simulink model "three_H_bridge"  (R2022b)
settings: Solver=FixedStepAuto  StartTime=0.0  StopTime=0.1  FixedStep=1e-7  MaxStep=1e-6  RelTol=5e-6
InitFcn:
  | fs=5000;
  | t1=(1/(3*fs));%模块内的载波时延
  | t2=(2/(3*fs));
  | m=1;
libraries: spsMosfetLib x72, spsSeriesRLCBranchLib x48, spsVoltageMeasurementLib x19, simulink x18, spsDCVoltageSourceLib x18, sps_lib x1
(part 1 of 2)
settings Model: Creator=zqf  LastModifiedBy=zqf

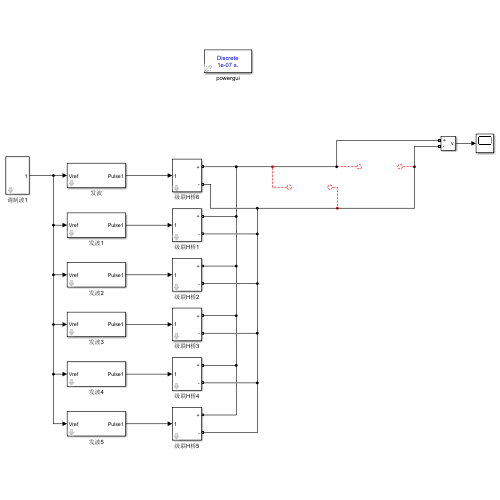
[thumbnail: Simulink's stored preview of the top-level diagram]
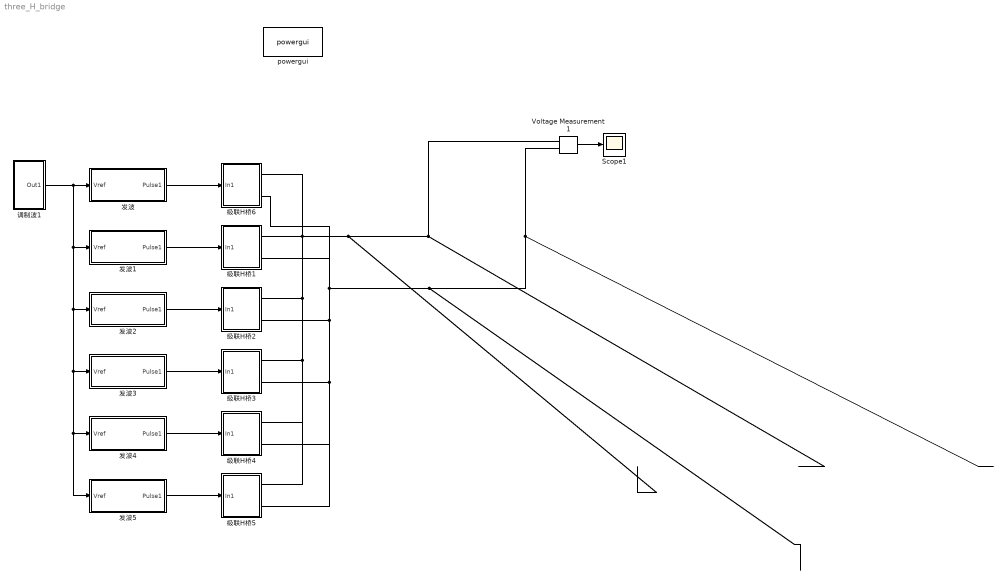
== system three_H_bridge ==
  Scope1 : Scope
  Voltage Measurement1 : spsVoltageMeasurementLib/Voltage Measurement  PhasorSimulation=off  OutputType=Complex  PSBequivalent=0
  powergui : sps_lib/powergui  Priority=1  SimulationMode=Discrete  SampleTime=1e-7  frequency=60  Iterations=50  frequencyindice=0  Pbase=100e6  ErrMax=1e-4  UnitsV=kV  UnitsW=MW  buscounter=0  FunctionMessages=off  echomessages=off  EnableUseOfTLC=off  CurrentSourceSwitches=off  DisableSnubberDevices=off  DisableRonSwitches=off  DisableVfSwitches=off  DisplayEquations=off  AutomaticDiscreteSolvers=off  SolverType=Tustin/Backward Euler (TBE)  Interpol=off  ExternalGateDelay=off  methode=off  Ts=100  x0status=blocks  SPID=on  SwTol=0  HookPort=off  NonlinearTolerance=1e-4  nMaxIteration=100  ContinueOnMaxIteration=off  RestoreLinks=warning  ResistiveCurrentMeasurement=off  Frange=[0:2:500]  Ylog=off  Xlog=on  ShowGrid=off  save=off  variable=ZData  structure=0  ZoomFFT=off  StartTime=0.0  cycles=1  DisplayStyle=1  fundamental=60  FreqAxis=off  MaxFrequency=1000  frequencyindicesteady=1  RmsSteady=1  display=off
  发波 : Subsystem  mask{n=0}
      mask prompts: n "延时n*Ts"
      mask DialogControl ParameterGroupVar Prompt: 参数
  发波1 : Subsystem  mask{n=(1/3)*(1/6)*m}
      mask prompts: n "延时n*Ts"
      mask DialogControl ParameterGroupVar Prompt: 参数
  发波2 : Subsystem  mask{n=(1/3)*(2/6)*m}
      mask prompts: n "延时n*Ts"
      mask DialogControl ParameterGroupVar Prompt: 参数
  发波3 : Subsystem  mask{n=(1/3)*(3/6)*m}
      mask prompts: n "延时n*Ts"
      mask DialogControl ParameterGroupVar Prompt: 参数
  发波4 : Subsystem  mask{n=(1/3)*(4/6)*m}
      mask prompts: n "延时n*Ts"
      mask DialogControl ParameterGroupVar Prompt: 参数
  发波5 : Subsystem  mask{n=(1/3)*(5/6)*m}
      mask prompts: n "延时n*Ts"
      mask DialogControl ParameterGroupVar Prompt: 参数
  级联H桥1 : Subsystem  mask{L=14E-6}
      mask DialogControl ParameterGroupVar Prompt: 参数
  级联H桥2 : Subsystem  mask{L=14E-6}
      mask DialogControl ParameterGroupVar Prompt: 参数
  级联H桥3 : Subsystem  mask{L=14E-6}
      mask DialogControl ParameterGroupVar Prompt: 参数
  级联H桥4 : Subsystem  mask{L=14E-6}
      mask DialogControl ParameterGroupVar Prompt: 参数
  级联H桥5 : Subsystem  mask{L=14E-6}
      mask DialogControl ParameterGroupVar Prompt: 参数
  级联H桥6 : Subsystem  mask{L=11E-6}
      mask DialogControl ParameterGroupVar Prompt: 参数
  调制波1 : Subsystem  mask{m=0.8}
      mask DialogControl ParameterGroupVar Prompt: 参数
  wires:
  发波3/1(Pulse1) -> 级联H桥3/1(In1)
  发波2/1(Pulse1) -> 级联H桥2/1(In1)
  Voltage Measurement1/1 -> Scope1/1
  发波5/1(Pulse1) -> 级联H桥5/1(In1)
  发波4/1(Pulse1) -> 级联H桥4/1(In1)
  发波/1(Pulse1) -> 级联H桥6/1(In1)
  调制波1/1(Out1) -> 发波1/1(Vref), 发波2/1(Vref), 发波3/1(Vref), 发波5/1(Vref), 发波4/1(Vref), 发波/1(Vref)
  发波1/1(Pulse1) -> 级联H桥1/1(In1)
  connections:
  级联H桥5/RConn2 -- 级联H桥4/RConn2 -- 级联H桥3/RConn2 -- 级联H桥2/RConn2 -- 级联H桥1/RConn2 -- Voltage Measurement1/LConn2 -- 级联H桥6/RConn2
  级联H桥5/RConn1 -- 级联H桥4/RConn1 -- 级联H桥3/RConn1 -- 级联H桥2/RConn1 -- 级联H桥1/RConn1 -- Voltage Measurement1/LConn1 -- 级联H桥6/RConn1

== system three_H_bridge/发波 ==
  Vref : Inport
  C+ : simulink/Sources/Repeating Sequence  rep_seq_t=[0 1/(2*fs) 1/(fs)]  rep_seq_y=[-1, 1, -1]
  C+2 : simulink/Sources/Repeating Sequence  rep_seq_t=[0 1/(2*fs) 1/(fs)]  rep_seq_y=[-1, 1, -1]
  C+3 : simulink/Sources/Repeating Sequence  rep_seq_t=[0 1/(2*fs) 1/(fs)]  rep_seq_y=[-1, 1, -1]
  Mux : Mux  Inputs=[4 4 4]
  Mux1 : Mux  Inputs=3
  Scope : Scope
  Scope2 : Scope  NumInputPorts=3
  Transport Delay : TransportDelay  DelayTime=t1
  Transport Delay1 : TransportDelay  DelayTime=t2
  Transport Delay2 : TransportDelay  DelayTime=n*(1/fs)
  Transport Delay3 : TransportDelay  DelayTime=n*(1/fs)
  Transport Delay4 : TransportDelay  DelayTime=n*(1/fs)
  单级倍频调制 : Subsystem
      settings: LibrarySourceBlock=|
      | powerlib_extras/Discrete
      | Control Blocks/Discrete 3-phase
      | PWM Generator/3-level Type/State-to-Pulses
      | Decoder
  单级倍频调制1 : Subsystem
      settings: LibrarySourceBlock=|
      | powerlib_extras/Discrete
      | Control Blocks/Discrete 3-phase
      | PWM Generator/3-level Type/State-to-Pulses
      | Decoder
  单级倍频调制2 : Subsystem
      settings: LibrarySourceBlock=|
      | powerlib_extras/Discrete
      | Control Blocks/Discrete 3-phase
      | PWM Generator/3-level Type/State-to-Pulses
      | Decoder
  Pulse1 : Outport
  wires:
  单级倍频调制2/1(Result) -> Mux/3
  单级倍频调制1/1(Result) -> Mux/2
  单级倍频调制/1(Result) -> Mux/1
  Vref/1 -> 单级倍频调制1/1(Modul), 单级倍频调制2/1(Modul), 单级倍频调制/1(Modul)
  Transport Delay/1 -> 单级倍频调制1/2(C+), Mux1/2, Scope2/2
  Transport Delay1/1 -> 单级倍频调制2/2(C+), Mux1/3, Scope2/3
  Mux/1 -> Pulse1/1
  Transport Delay3/1 -> Mux1/1, Scope2/1, 单级倍频调制/2(C+)
  C+/1 -> Transport Delay3/1
  C+2/1 -> Transport Delay2/1
  Transport Delay2/1 -> Transport Delay/1
  Transport Delay4/1 -> Transport Delay1/1
  C+3/1 -> Transport Delay4/1
  Mux1/1 -> Scope/1

== system three_H_bridge/发波1 ==
  Vref : Inport
  C+ : simulink/Sources/Repeating Sequence  rep_seq_t=[0 1/(2*fs) 1/(fs)]  rep_seq_y=[-1, 1, -1]
  C+2 : simulink/Sources/Repeating Sequence  rep_seq_t=[0 1/(2*fs) 1/(fs)]  rep_seq_y=[-1, 1, -1]
  C+3 : simulink/Sources/Repeating Sequence  rep_seq_t=[0 1/(2*fs) 1/(fs)]  rep_seq_y=[-1, 1, -1]
  Mux : Mux  Inputs=[4 4 4]
  Mux1 : Mux  Inputs=3
  Scope : Scope
  Scope2 : Scope  NumInputPorts=3
  Transport Delay : TransportDelay  DelayTime=t1
  Transport Delay1 : TransportDelay  DelayTime=t2
  Transport Delay2 : TransportDelay  DelayTime=n*(1/fs)
  Transport Delay3 : TransportDelay  DelayTime=n*(1/fs)
  Transport Delay4 : TransportDelay  DelayTime=n*(1/fs)
  单级倍频调制 : Subsystem
      settings: LibrarySourceBlock=|
      | powerlib_extras/Discrete
      | Control Blocks/Discrete 3-phase
      | PWM Generator/3-level Type/State-to-Pulses
      | Decoder
  单级倍频调制1 : Subsystem
      settings: LibrarySourceBlock=|
      | powerlib_extras/Discrete
      | Control Blocks/Discrete 3-phase
      | PWM Generator/3-level Type/State-to-Pulses
      | Decoder
  单级倍频调制2 : Subsystem
      settings: LibrarySourceBlock=|
      | powerlib_extras/Discrete
      | Control Blocks/Discrete 3-phase
      | PWM Generator/3-level Type/State-to-Pulses
      | Decoder
  Pulse1 : Outport
  wires:
  Mux1/1 -> Scope/1
  C+3/1 -> Transport Delay4/1
  Transport Delay4/1 -> Transport Delay1/1
  Transport Delay2/1 -> Transport Delay/1
  C+2/1 -> Transport Delay2/1
  C+/1 -> Transport Delay3/1
  Transport Delay3/1 -> 单级倍频调制/2(C+), Scope2/1, Mux1/1
  Mux/1 -> Pulse1/1
  Transport Delay1/1 -> Scope2/3, Mux1/3, 单级倍频调制2/2(C+)
  Transport Delay/1 -> Scope2/2, Mux1/2, 单级倍频调制1/2(C+)
  Vref/1 -> 单级倍频调制/1(Modul), 单级倍频调制2/1(Modul), 单级倍频调制1/1(Modul)
  单级倍频调制/1(Result) -> Mux/1
  单级倍频调制1/1(Result) -> Mux/2
  单级倍频调制2/1(Result) -> Mux/3

== system three_H_bridge/发波2 ==
  Vref : Inport
  C+ : simulink/Sources/Repeating Sequence  rep_seq_t=[0 1/(2*fs) 1/(fs)]  rep_seq_y=[-1, 1, -1]
  C+2 : simulink/Sources/Repeating Sequence  rep_seq_t=[0 1/(2*fs) 1/(fs)]  rep_seq_y=[-1, 1, -1]
  C+3 : simulink/Sources/Repeating Sequence  rep_seq_t=[0 1/(2*fs) 1/(fs)]  rep_seq_y=[-1, 1, -1]
  Mux : Mux  Inputs=[4 4 4]
  Mux1 : Mux  Inputs=3
  Scope : Scope
  Scope2 : Scope  NumInputPorts=3
  Transport Delay : TransportDelay  DelayTime=t1
  Transport Delay1 : TransportDelay  DelayTime=t2
  Transport Delay2 : TransportDelay  DelayTime=n*(1/fs)
  Transport Delay3 : TransportDelay  DelayTime=n*(1/fs)
  Transport Delay4 : TransportDelay  DelayTime=n*(1/fs)
  单级倍频调制 : Subsystem
      settings: LibrarySourceBlock=|
      | powerlib_extras/Discrete
      | Control Blocks/Discrete 3-phase
      | PWM Generator/3-level Type/State-to-Pulses
      | Decoder
  单级倍频调制1 : Subsystem
      settings: LibrarySourceBlock=|
      | powerlib_extras/Discrete
      | Control Blocks/Discrete 3-phase
      | PWM Generator/3-level Type/State-to-Pulses
      | Decoder
  单级倍频调制2 : Subsystem
      settings: LibrarySourceBlock=|
      | powerlib_extras/Discrete
      | Control Blocks/Discrete 3-phase
      | PWM Generator/3-level Type/State-to-Pulses
      | Decoder
  Pulse1 : Outport
  wires:
  单级倍频调制2/1(Result) -> Mux/3
  单级倍频调制1/1(Result) -> Mux/2
  单级倍频调制/1(Result) -> Mux/1
  Vref/1 -> 单级倍频调制1/1(Modul), 单级倍频调制2/1(Modul), 单级倍频调制/1(Modul)
  Transport Delay/1 -> 单级倍频调制1/2(C+), Mux1/2, Scope2/2
  Transport Delay1/1 -> 单级倍频调制2/2(C+), Mux1/3, Scope2/3
  Mux/1 -> Pulse1/1
  Transport Delay3/1 -> Mux1/1, Scope2/1, 单级倍频调制/2(C+)
  C+/1 -> Transport Delay3/1
  C+2/1 -> Transport Delay2/1
  Transport Delay2/1 -> Transport Delay/1
  Transport Delay4/1 -> Transport Delay1/1
  C+3/1 -> Transport Delay4/1
  Mux1/1 -> Scope/1

== system three_H_bridge/发波3 ==
  Vref : Inport
  C+ : simulink/Sources/Repeating Sequence  rep_seq_t=[0 1/(2*fs) 1/(fs)]  rep_seq_y=[-1, 1, -1]
  C+2 : simulink/Sources/Repeating Sequence  rep_seq_t=[0 1/(2*fs) 1/(fs)]  rep_seq_y=[-1, 1, -1]
  C+3 : simulink/Sources/Repeating Sequence  rep_seq_t=[0 1/(2*fs) 1/(fs)]  rep_seq_y=[-1, 1, -1]
  Mux : Mux  Inputs=[4 4 4]
  Mux1 : Mux  Inputs=3
  Scope : Scope
  Scope2 : Scope  NumInputPorts=3
  Transport Delay : TransportDelay  DelayTime=t1
  Transport Delay1 : TransportDelay  DelayTime=t2
  Transport Delay2 : TransportDelay  DelayTime=n*(1/fs)
  Transport Delay3 : TransportDelay  DelayTime=n*(1/fs)
  Transport Delay4 : TransportDelay  DelayTime=n*(1/fs)
  单级倍频调制 : Subsystem
      settings: LibrarySourceBlock=|
      | powerlib_extras/Discrete
      | Control Blocks/Discrete 3-phase
      | PWM Generator/3-level Type/State-to-Pulses
      | Decoder
  单级倍频调制1 : Subsystem
      settings: LibrarySourceBlock=|
      | powerlib_extras/Discrete
      | Control Blocks/Discrete 3-phase
      | PWM Generator/3-level Type/State-to-Pulses
      | Decoder
  单级倍频调制2 : Subsystem
      settings: LibrarySourceBlock=|
      | powerlib_extras/Discrete
      | Control Blocks/Discrete 3-phase
      | PWM Generator/3-level Type/State-to-Pulses
      | Decoder
  Pulse1 : Outport
  wires:
  Mux1/1 -> Scope/1
  C+3/1 -> Transport Delay4/1
  Transport Delay4/1 -> Transport Delay1/1
  Transport Delay2/1 -> Transport Delay/1
  C+2/1 -> Transport Delay2/1
  C+/1 -> Transport Delay3/1
  Transport Delay3/1 -> 单级倍频调制/2(C+), Scope2/1, Mux1/1
  Mux/1 -> Pulse1/1
  Transport Delay1/1 -> Scope2/3, Mux1/3, 单级倍频调制2/2(C+)
  Transport Delay/1 -> Scope2/2, Mux1/2, 单级倍频调制1/2(C+)
  Vref/1 -> 单级倍频调制/1(Modul), 单级倍频调制2/1(Modul), 单级倍频调制1/1(Modul)
  单级倍频调制/1(Result) -> Mux/1
  单级倍频调制1/1(Result) -> Mux/2
  单级倍频调制2/1(Result) -> Mux/3

== system three_H_bridge/发波4 ==
  Vref : Inport
  C+ : simulink/Sources/Repeating Sequence  rep_seq_t=[0 1/(2*fs) 1/(fs)]  rep_seq_y=[-1, 1, -1]
  C+2 : simulink/Sources/Repeating Sequence  rep_seq_t=[0 1/(2*fs) 1/(fs)]  rep_seq_y=[-1, 1, -1]
  C+3 : simulink/Sources/Repeating Sequence  rep_seq_t=[0 1/(2*fs) 1/(fs)]  rep_seq_y=[-1, 1, -1]
  Mux : Mux  Inputs=[4 4 4]
  Mux1 : Mux  Inputs=3
  Scope : Scope
  Scope2 : Scope  NumInputPorts=3
  Transport Delay : TransportDelay  DelayTime=t1
  Transport Delay1 : TransportDelay  DelayTime=t2
  Transport Delay2 : TransportDelay  DelayTime=n*(1/fs)
  Transport Delay3 : TransportDelay  DelayTime=n*(1/fs)
  Transport Delay4 : TransportDelay  DelayTime=n*(1/fs)
  单级倍频调制 : Subsystem
      settings: LibrarySourceBlock=|
      | powerlib_extras/Discrete
      | Control Blocks/Discrete 3-phase
      | PWM Generator/3-level Type/State-to-Pulses
      | Decoder
  单级倍频调制1 : Subsystem
      settings: LibrarySourceBlock=|
      | powerlib_extras/Discrete
      | Control Blocks/Discrete 3-phase
      | PWM Generator/3-level Type/State-to-Pulses
      | Decoder
  单级倍频调制2 : Subsystem
      settings: LibrarySourceBlock=|
      | powerlib_extras/Discrete
      | Control Blocks/Discrete 3-phase
      | PWM Generator/3-level Type/State-to-Pulses
      | Decoder
  Pulse1 : Outport
  wires:
  单级倍频调制2/1(Result) -> Mux/3
  单级倍频调制1/1(Result) -> Mux/2
  单级倍频调制/1(Result) -> Mux/1
  Vref/1 -> 单级倍频调制1/1(Modul), 单级倍频调制2/1(Modul), 单级倍频调制/1(Modul)
  Transport Delay/1 -> 单级倍频调制1/2(C+), Mux1/2, Scope2/2
  Transport Delay1/1 -> 单级倍频调制2/2(C+), Mux1/3, Scope2/3
  Mux/1 -> Pulse1/1
  Transport Delay3/1 -> Mux1/1, Scope2/1, 单级倍频调制/2(C+)
  C+/1 -> Transport Delay3/1
  C+2/1 -> Transport Delay2/1
  Transport Delay2/1 -> Transport Delay/1
  Transport Delay4/1 -> Transport Delay1/1
  C+3/1 -> Transport Delay4/1
  Mux1/1 -> Scope/1

== system three_H_bridge/发波5 ==
  Vref : Inport
  C+ : simulink/Sources/Repeating Sequence  rep_seq_t=[0 1/(2*fs) 1/(fs)]  rep_seq_y=[-1, 1, -1]
  C+2 : simulink/Sources/Repeating Sequence  rep_seq_t=[0 1/(2*fs) 1/(fs)]  rep_seq_y=[-1, 1, -1]
  C+3 : simulink/Sources/Repeating Sequence  rep_seq_t=[0 1/(2*fs) 1/(fs)]  rep_seq_y=[-1, 1, -1]
  Mux : Mux  Inputs=[4 4 4]
  Mux1 : Mux  Inputs=3
  Scope : Scope
  Scope2 : Scope  NumInputPorts=3
  Transport Delay : TransportDelay  DelayTime=t1
  Transport Delay1 : TransportDelay  DelayTime=t2
  Transport Delay2 : TransportDelay  DelayTime=n*(1/fs)
  Transport Delay3 : TransportDelay  DelayTime=n*(1/fs)
  Transport Delay4 : TransportDelay  DelayTime=n*(1/fs)
  单级倍频调制 : Subsystem
      settings: LibrarySourceBlock=|
      | powerlib_extras/Discrete
      | Control Blocks/Discrete 3-phase
      | PWM Generator/3-level Type/State-to-Pulses
      | Decoder
  单级倍频调制1 : Subsystem
      settings: LibrarySourceBlock=|
      | powerlib_extras/Discrete
      | Control Blocks/Discrete 3-phase
      | PWM Generator/3-level Type/State-to-Pulses
      | Decoder
  单级倍频调制2 : Subsystem
      settings: LibrarySourceBlock=|
      | powerlib_extras/Discrete
      | Control Blocks/Discrete 3-phase
      | PWM Generator/3-level Type/State-to-Pulses
      | Decoder
  Pulse1 : Outport
  wires:
  Mux1/1 -> Scope/1
  C+3/1 -> Transport Delay4/1
  Transport Delay4/1 -> Transport Delay1/1
  Transport Delay2/1 -> Transport Delay/1
  C+2/1 -> Transport Delay2/1
  C+/1 -> Transport Delay3/1
  Transport Delay3/1 -> 单级倍频调制/2(C+), Scope2/1, Mux1/1
  Mux/1 -> Pulse1/1
  Transport Delay1/1 -> Scope2/3, Mux1/3, 单级倍频调制2/2(C+)
  Transport Delay/1 -> Scope2/2, Mux1/2, 单级倍频调制1/2(C+)
  Vref/1 -> 单级倍频调制/1(Modul), 单级倍频调制2/1(Modul), 单级倍频调制1/1(Modul)
  单级倍频调制/1(Result) -> Mux/1
  单级倍频调制1/1(Result) -> Mux/2
  单级倍频调制2/1(Result) -> Mux/3

== system three_H_bridge/级联H桥1 ==
  In1 : Inport
  Demux : Demux  Outputs=[4 4 4]
  H桥 : Subsystem
  H桥1 : Subsystem
  H桥2 : Subsystem
  Series RLC Branch6 : spsSeriesRLCBranchLib/Series RLC Branch  LConnTagsString=__new0  RConnTagsString=__new0  BranchType=L  Resistance=1  Inductance=L  SetiL0=off  InitialCurrent=0  Capacitance=1e-6  Setx0=off  InitialVoltage=0  Measurements=None
  Series RLC Branch7 : spsSeriesRLCBranchLib/Series RLC Branch  LConnTagsString=__new0  RConnTagsString=__new0  BranchType=L  Resistance=1  Inductance=L  SetiL0=off  InitialCurrent=0  Capacitance=1e-6  Setx0=off  InitialVoltage=0  Measurements=None
  + : PMIOPort  Side=Right
  - : PMIOPort  Port=2  Side=Right
  wires:
  Demux/3 -> H桥2/1(In1)
  Demux/2 -> H桥1/1(In1)
  Demux/1 -> H桥/1(In1)
  In1/1 -> Demux/1
  connections:
  H桥1/RConn1 -- H桥/RConn2
  H桥2/RConn2 -- Series RLC Branch7/LConn1
  H桥2/RConn1 -- H桥1/RConn2
  Series RLC Branch6/LConn1 -- H桥/RConn1
  +/RConn1 -- Series RLC Branch6/RConn1
  -/RConn1 -- Series RLC Branch7/RConn1

== system three_H_bridge/级联H桥2 ==
  In1 : Inport
  Demux : Demux  Outputs=[4 4 4]
  H桥 : Subsystem
  H桥1 : Subsystem
  H桥2 : Subsystem
  Series RLC Branch6 : spsSeriesRLCBranchLib/Series RLC Branch  LConnTagsString=__new0  RConnTagsString=__new0  BranchType=L  Resistance=1  Inductance=L  SetiL0=off  InitialCurrent=0  Capacitance=1e-6  Setx0=off  InitialVoltage=0  Measurements=None
  Series RLC Branch7 : spsSeriesRLCBranchLib/Series RLC Branch  LConnTagsString=__new0  RConnTagsString=__new0  BranchType=L  Resistance=1  Inductance=L  SetiL0=off  InitialCurrent=0  Capacitance=1e-6  Setx0=off  InitialVoltage=0  Measurements=None
  + : PMIOPort  Side=Right
  - : PMIOPort  Port=2  Side=Right
  wires:
  In1/1 -> Demux/1
  Demux/1 -> H桥/1(In1)
  Demux/2 -> H桥1/1(In1)
  Demux/3 -> H桥2/1(In1)
  connections:
  -/RConn1 -- Series RLC Branch7/RConn1
  +/RConn1 -- Series RLC Branch6/RConn1
  Series RLC Branch6/LConn1 -- H桥/RConn1
  H桥2/RConn1 -- H桥1/RConn2
  H桥2/RConn2 -- Series RLC Branch7/LConn1
  H桥1/RConn1 -- H桥/RConn2

== system three_H_bridge/级联H桥3 ==
  In1 : Inport
  Demux : Demux  Outputs=[4 4 4]
  H桥 : Subsystem
  H桥1 : Subsystem
  H桥2 : Subsystem
  Series RLC Branch6 : spsSeriesRLCBranchLib/Series RLC Branch  LConnTagsString=__new0  RConnTagsString=__new0  BranchType=L  Resistance=1  Inductance=L  SetiL0=off  InitialCurrent=0  Capacitance=1e-6  Setx0=off  InitialVoltage=0  Measurements=None
  Series RLC Branch7 : spsSeriesRLCBranchLib/Series RLC Branch  LConnTagsString=__new0  RConnTagsString=__new0  BranchType=L  Resistance=1  Inductance=L  SetiL0=off  InitialCurrent=0  Capacitance=1e-6  Setx0=off  InitialVoltage=0  Measurements=None
  + : PMIOPort  Side=Right
  - : PMIOPort  Port=2  Side=Right
  wires:
  Demux/3 -> H桥2/1(In1)
  Demux/2 -> H桥1/1(In1)
  Demux/1 -> H桥/1(In1)
  In1/1 -> Demux/1
  connections:
  H桥1/RConn1 -- H桥/RConn2
  H桥2/RConn2 -- Series RLC Branch7/LConn1
  H桥2/RConn1 -- H桥1/RConn2
  Series RLC Branch6/LConn1 -- H桥/RConn1
  +/RConn1 -- Series RLC Branch6/RConn1
  -/RConn1 -- Series RLC Branch7/RConn1

== system three_H_bridge/级联H桥4 ==
  In1 : Inport
  Demux : Demux  Outputs=[4 4 4]
  H桥 : Subsystem
  H桥1 : Subsystem
  H桥2 : Subsystem
  Series RLC Branch6 : spsSeriesRLCBranchLib/Series RLC Branch  LConnTagsString=__new0  RConnTagsString=__new0  BranchType=L  Resistance=1  Inductance=L  SetiL0=off  InitialCurrent=0  Capacitance=1e-6  Setx0=off  InitialVoltage=0  Measurements=None
  Series RLC Branch7 : spsSeriesRLCBranchLib/Series RLC Branch  LConnTagsString=__new0  RConnTagsString=__new0  BranchType=L  Resistance=1  Inductance=L  SetiL0=off  InitialCurrent=0  Capacitance=1e-6  Setx0=off  InitialVoltage=0  Measurements=None
  + : PMIOPort  Side=Right
  - : PMIOPort  Port=2  Side=Right
  wires:
  In1/1 -> Demux/1
  Demux/1 -> H桥/1(In1)
  Demux/2 -> H桥1/1(In1)
  Demux/3 -> H桥2/1(In1)
  connections:
  -/RConn1 -- Series RLC Branch7/RConn1
  +/RConn1 -- Series RLC Branch6/RConn1
  Series RLC Branch6/LConn1 -- H桥/RConn1
  H桥2/RConn1 -- H桥1/RConn2
  H桥2/RConn2 -- Series RLC Branch7/LConn1
  H桥1/RConn1 -- H桥/RConn2

== system three_H_bridge/级联H桥5 ==
  In1 : Inport
  Demux : Demux  Outputs=[4 4 4]
  H桥 : Subsystem
  H桥1 : Subsystem
  H桥2 : Subsystem
  Series RLC Branch6 : spsSeriesRLCBranchLib/Series RLC Branch  LConnTagsString=__new0  RConnTagsString=__new0  BranchType=L  Resistance=1  Inductance=L  SetiL0=off  InitialCurrent=0  Capacitance=1e-6  Setx0=off  InitialVoltage=0  Measurements=None
  Series RLC Branch7 : spsSeriesRLCBranchLib/Series RLC Branch  LConnTagsString=__new0  RConnTagsString=__new0  BranchType=L  Resistance=1  Inductance=L  SetiL0=off  InitialCurrent=0  Capacitance=1e-6  Setx0=off  InitialVoltage=0  Measurements=None
  + : PMIOPort  Side=Right
  - : PMIOPort  Port=2  Side=Right
  wires:
  Demux/3 -> H桥2/1(In1)
  Demux/2 -> H桥1/1(In1)
  Demux/1 -> H桥/1(In1)
  In1/1 -> Demux/1
  connections:
  H桥1/RConn1 -- H桥/RConn2
  H桥2/RConn2 -- Series RLC Branch7/LConn1
  H桥2/RConn1 -- H桥1/RConn2
  Series RLC Branch6/LConn1 -- H桥/RConn1
  +/RConn1 -- Series RLC Branch6/RConn1
  -/RConn1 -- Series RLC Branch7/RConn1

== system three_H_bridge/级联H桥6 ==
  In1 : Inport
  Demux : Demux  Outputs=[4 4 4]
  H桥 : Subsystem
  H桥1 : Subsystem
  H桥2 : Subsystem
  Series RLC Branch6 : spsSeriesRLCBranchLib/Series RLC Branch  LConnTagsString=__new0  RConnTagsString=__new0  BranchType=L  Resistance=1  Inductance=L  SetiL0=off  InitialCurrent=0  Capacitance=1e-6  Setx0=off  InitialVoltage=0  Measurements=None
  Series RLC Branch7 : spsSeriesRLCBranchLib/Series RLC Branch  LConnTagsString=__new0  RConnTagsString=__new0  BranchType=L  Resistance=1  Inductance=L  SetiL0=off  InitialCurrent=0  Capacitance=1e-6  Setx0=off  InitialVoltage=0  Measurements=None
  + : PMIOPort  Side=Right
  - : PMIOPort  Port=2  Side=Right
  wires:
  In1/1 -> Demux/1
  Demux/1 -> H桥/1(In1)
  Demux/2 -> H桥1/1(In1)
  Demux/3 -> H桥2/1(In1)
  connections:
  -/RConn1 -- Series RLC Branch7/RConn1
  +/RConn1 -- Series RLC Branch6/RConn1
  Series RLC Branch6/LConn1 -- H桥/RConn1
  H桥2/RConn1 -- H桥1/RConn2
  H桥2/RConn2 -- Series RLC Branch7/LConn1
  H桥1/RConn1 -- H桥/RConn2

== system three_H_bridge/调制波1 ==
  Mux : Mux  Commented=on  Inputs=3
  Sine Wave : Sin  Amplitude=m  Frequency=50/(1/(2*pi))  SampleTime=0
  Sine Wave1 : Sin  Commented=on  Amplitude=m  Frequency=50/(1/(2*pi))  Phase=(120/180)*pi  SampleTime=0
  Sine Wave2 : Sin  Commented=on  Amplitude=m  Frequency=50/(1/(2*pi))  Phase=(-120/180)*pi  SampleTime=0
  Out1 : Outport
  wires:
  Sine Wave2/1 -> Mux/3
  Sine Wave1/1 -> Mux/2
  Sine Wave/1 -> Out1/1, Mux/1

== system three_H_bridge/发波/单级倍频调制 ==
  note: 1
  Modul : Inport  PortDimensions=1
  C+ : Inport  Port=2  PortDimensions=1
  Constant : Constant  Value=-1
  Logical Operator : Logic  Operator=NOT  AllPortsSameDT=off  OutDataTypeStr=boolean
  Logical Operator1 : Logic  Operator=NOT  AllPortsSameDT=off  OutDataTypeStr=boolean
  Mux : Mux
  Product : Product
  Relational Operator1 : RelationalOperator  OutDataTypeStr=boolean  InputSameDT=off
  Relational Operator2 : RelationalOperator  OutDataTypeStr=boolean  InputSameDT=off
  Result : Outport
  wires:
  C+/1 -> Relational Operator2/2, Product/1
  Modul/1 -> Relational Operator1/1, Relational Operator2/1
  Relational Operator2/1 -> Logical Operator/1, Mux/1
  Logical Operator/1 -> Mux/2
  Constant/1 -> Product/2
  Product/1 -> Relational Operator1/2
  Mux/1 -> Result/1
  Relational Operator1/1 -> Logical Operator1/1, Mux/4
  Logical Operator1/1 -> Mux/3

== system three_H_bridge/发波/单级倍频调制1 ==
  note: 1
  Modul : Inport  PortDimensions=1
  C+ : Inport  Port=2  PortDimensions=1
  Constant : Constant  Value=-1
  Logical Operator : Logic  Operator=NOT  AllPortsSameDT=off  OutDataTypeStr=boolean
  Logical Operator1 : Logic  Operator=NOT  AllPortsSameDT=off  OutDataTypeStr=boolean
  Mux : Mux
  Product : Product
  Relational Operator1 : RelationalOperator  OutDataTypeStr=boolean  InputSameDT=off
  Relational Operator2 : RelationalOperator  OutDataTypeStr=boolean  InputSameDT=off
  Result : Outport
  wires:
  Logical Operator1/1 -> Mux/3
  Relational Operator1/1 -> Mux/4, Logical Operator1/1
  Mux/1 -> Result/1
  Product/1 -> Relational Operator1/2
  Constant/1 -> Product/2
  Logical Operator/1 -> Mux/2
  Relational Operator2/1 -> Mux/1, Logical Operator/1
  Modul/1 -> Relational Operator2/1, Relational Operator1/1
  C+/1 -> Product/1, Relational Operator2/2

== system three_H_bridge/发波/单级倍频调制2 ==
  note: 1
  Modul : Inport  PortDimensions=1
  C+ : Inport  Port=2  PortDimensions=1
  Constant : Constant  Value=-1
  Logical Operator : Logic  Operator=NOT  AllPortsSameDT=off  OutDataTypeStr=boolean
  Logical Operator1 : Logic  Operator=NOT  AllPortsSameDT=off  OutDataTypeStr=boolean
  Mux : Mux
  Product : Product
  Relational Operator1 : RelationalOperator  OutDataTypeStr=boolean  InputSameDT=off
  Relational Operator2 : RelationalOperator  OutDataTypeStr=boolean  InputSameDT=off
  Result : Outport
  wires:
  C+/1 -> Relational Operator2/2, Product/1
  Modul/1 -> Relational Operator1/1, Relational Operator2/1
  Relational Operator2/1 -> Logical Operator/1, Mux/1
  Logical Operator/1 -> Mux/2
  Constant/1 -> Product/2
  Product/1 -> Relational Operator1/2
  Mux/1 -> Result/1
  Relational Operator1/1 -> Logical Operator1/1, Mux/4
  Logical Operator1/1 -> Mux/3

== system three_H_bridge/发波1/单级倍频调制 ==
  note: 1
  Modul : Inport  PortDimensions=1
  C+ : Inport  Port=2  PortDimensions=1
  Constant : Constant  Value=-1
  Logical Operator : Logic  Operator=NOT  AllPortsSameDT=off  OutDataTypeStr=boolean
  Logical Operator1 : Logic  Operator=NOT  AllPortsSameDT=off  OutDataTypeStr=boolean
  Mux : Mux
  Product : Product
  Relational Operator1 : RelationalOperator  OutDataTypeStr=boolean  InputSameDT=off
  Relational Operator2 : RelationalOperator  OutDataTypeStr=boolean  InputSameDT=off
  Result : Outport
  wires:
  Logical Operator1/1 -> Mux/3
  Relational Operator1/1 -> Mux/4, Logical Operator1/1
  Mux/1 -> Result/1
  Product/1 -> Relational Operator1/2
  Constant/1 -> Product/2
  Logical Operator/1 -> Mux/2
  Relational Operator2/1 -> Mux/1, Logical Operator/1
  Modul/1 -> Relational Operator2/1, Relational Operator1/1
  C+/1 -> Product/1, Relational Operator2/2

== system three_H_bridge/发波1/单级倍频调制1 ==
  note: 1
  Modul : Inport  PortDimensions=1
  C+ : Inport  Port=2  PortDimensions=1
  Constant : Constant  Value=-1
  Logical Operator : Logic  Operator=NOT  AllPortsSameDT=off  OutDataTypeStr=boolean
  Logical Operator1 : Logic  Operator=NOT  AllPortsSameDT=off  OutDataTypeStr=boolean
  Mux : Mux
  Product : Product
  Relational Operator1 : RelationalOperator  OutDataTypeStr=boolean  InputSameDT=off
  Relational Operator2 : RelationalOperator  OutDataTypeStr=boolean  InputSameDT=off
  Result : Outport
  wires:
  C+/1 -> Relational Operator2/2, Product/1
  Modul/1 -> Relational Operator1/1, Relational Operator2/1
  Relational Operator2/1 -> Logical Operator/1, Mux/1
  Logical Operator/1 -> Mux/2
  Constant/1 -> Product/2
  Product/1 -> Relational Operator1/2
  Mux/1 -> Result/1
  Relational Operator1/1 -> Logical Operator1/1, Mux/4
  Logical Operator1/1 -> Mux/3

== system three_H_bridge/发波1/单级倍频调制2 ==
  note: 1
  Modul : Inport  PortDimensions=1
  C+ : Inport  Port=2  PortDimensions=1
  Constant : Constant  Value=-1
  Logical Operator : Logic  Operator=NOT  AllPortsSameDT=off  OutDataTypeStr=boolean
  Logical Operator1 : Logic  Operator=NOT  AllPortsSameDT=off  OutDataTypeStr=boolean
  Mux : Mux
  Product : Product
  Relational Operator1 : RelationalOperator  OutDataTypeStr=boolean  InputSameDT=off
  Relational Operator2 : RelationalOperator  OutDataTypeStr=boolean  InputSameDT=off
  Result : Outport
  wires:
  Logical Operator1/1 -> Mux/3
  Relational Operator1/1 -> Mux/4, Logical Operator1/1
  Mux/1 -> Result/1
  Product/1 -> Relational Operator1/2
  Constant/1 -> Product/2
  Logical Operator/1 -> Mux/2
  Relational Operator2/1 -> Mux/1, Logical Operator/1
  Modul/1 -> Relational Operator2/1, Relational Operator1/1
  C+/1 -> Product/1, Relational Operator2/2

== system three_H_bridge/发波2/单级倍频调制 ==
  note: 1
  Modul : Inport  PortDimensions=1
  C+ : Inport  Port=2  PortDimensions=1
  Constant : Constant  Value=-1
  Logical Operator : Logic  Operator=NOT  AllPortsSameDT=off  OutDataTypeStr=boolean
  Logical Operator1 : Logic  Operator=NOT  AllPortsSameDT=off  OutDataTypeStr=boolean
  Mux : Mux
  Product : Product
  Relational Operator1 : RelationalOperator  OutDataTypeStr=boolean  InputSameDT=off
  Relational Operator2 : RelationalOperator  OutDataTypeStr=boolean  InputSameDT=off
  Result : Outport
  wires:
  C+/1 -> Relational Operator2/2, Product/1
  Modul/1 -> Relational Operator1/1, Relational Operator2/1
  Relational Operator2/1 -> Logical Operator/1, Mux/1
  Logical Operator/1 -> Mux/2
  Constant/1 -> Product/2
  Product/1 -> Relational Operator1/2
  Mux/1 -> Result/1
  Relational Operator1/1 -> Logical Operator1/1, Mux/4
  Logical Operator1/1 -> Mux/3

== system three_H_bridge/发波2/单级倍频调制1 ==
  note: 1
  Modul : Inport  PortDimensions=1
  C+ : Inport  Port=2  PortDimensions=1
  Constant : Constant  Value=-1
  Logical Operator : Logic  Operator=NOT  AllPortsSameDT=off  OutDataTypeStr=boolean
  Logical Operator1 : Logic  Operator=NOT  AllPortsSameDT=off  OutDataTypeStr=boolean
  Mux : Mux
  Product : Product
  Relational Operator1 : RelationalOperator  OutDataTypeStr=boolean  InputSameDT=off
  Relational Operator2 : RelationalOperator  OutDataTypeStr=boolean  InputSameDT=off
  Result : Outport
  wires:
  Logical Operator1/1 -> Mux/3
  Relational Operator1/1 -> Mux/4, Logical Operator1/1
  Mux/1 -> Result/1
  Product/1 -> Relational Operator1/2
  Constant/1 -> Product/2
  Logical Operator/1 -> Mux/2
  Relational Operator2/1 -> Mux/1, Logical Operator/1
  Modul/1 -> Relational Operator2/1, Relational Operator1/1
  C+/1 -> Product/1, Relational Operator2/2

== system three_H_bridge/发波2/单级倍频调制2 ==
  note: 1
  Modul : Inport  PortDimensions=1
  C+ : Inport  Port=2  PortDimensions=1
  Constant : Constant  Value=-1
  Logical Operator : Logic  Operator=NOT  AllPortsSameDT=off  OutDataTypeStr=boolean
  Logical Operator1 : Logic  Operator=NOT  AllPortsSameDT=off  OutDataTypeStr=boolean
  Mux : Mux
  Product : Product
  Relational Operator1 : RelationalOperator  OutDataTypeStr=boolean  InputSameDT=off
  Relational Operator2 : RelationalOperator  OutDataTypeStr=boolean  InputSameDT=off
  Result : Outport
  wires:
  C+/1 -> Relational Operator2/2, Product/1
  Modul/1 -> Relational Operator1/1, Relational Operator2/1
  Relational Operator2/1 -> Logical Operator/1, Mux/1
  Logical Operator/1 -> Mux/2
  Constant/1 -> Product/2
  Product/1 -> Relational Operator1/2
  Mux/1 -> Result/1
  Relational Operator1/1 -> Logical Operator1/1, Mux/4
  Logical Operator1/1 -> Mux/3

== system three_H_bridge/发波3/单级倍频调制 ==
  note: 1
  Modul : Inport  PortDimensions=1
  C+ : Inport  Port=2  PortDimensions=1
  Constant : Constant  Value=-1
  Logical Operator : Logic  Operator=NOT  AllPortsSameDT=off  OutDataTypeStr=boolean
  Logical Operator1 : Logic  Operator=NOT  AllPortsSameDT=off  OutDataTypeStr=boolean
  Mux : Mux
  Product : Product
  Relational Operator1 : RelationalOperator  OutDataTypeStr=boolean  InputSameDT=off
  Relational Operator2 : RelationalOperator  OutDataTypeStr=boolean  InputSameDT=off
  Result : Outport
  wires:
  Logical Operator1/1 -> Mux/3
  Relational Operator1/1 -> Mux/4, Logical Operator1/1
  Mux/1 -> Result/1
  Product/1 -> Relational Operator1/2
  Constant/1 -> Product/2
  Logical Operator/1 -> Mux/2
  Relational Operator2/1 -> Mux/1, Logical Operator/1
  Modul/1 -> Relational Operator2/1, Relational Operator1/1
  C+/1 -> Product/1, Relational Operator2/2

== system three_H_bridge/发波3/单级倍频调制1 ==
  note: 1
  Modul : Inport  PortDimensions=1
  C+ : Inport  Port=2  PortDimensions=1
  Constant : Constant  Value=-1
  Logical Operator : Logic  Operator=NOT  AllPortsSameDT=off  OutDataTypeStr=boolean
  Logical Operator1 : Logic  Operator=NOT  AllPortsSameDT=off  OutDataTypeStr=boolean
  Mux : Mux
  Product : Product
  Relational Operator1 : RelationalOperator  OutDataTypeStr=boolean  InputSameDT=off
  Relational Operator2 : RelationalOperator  OutDataTypeStr=boolean  InputSameDT=off
  Result : Outport
  wires:
  C+/1 -> Relational Operator2/2, Product/1
  Modul/1 -> Relational Operator1/1, Relational Operator2/1
  Relational Operator2/1 -> Logical Operator/1, Mux/1
  Logical Operator/1 -> Mux/2
  Constant/1 -> Product/2
  Product/1 -> Relational Operator1/2
  Mux/1 -> Result/1
  Relational Operator1/1 -> Logical Operator1/1, Mux/4
  Logical Operator1/1 -> Mux/3

== system three_H_bridge/发波3/单级倍频调制2 ==
  note: 1
  Modul : Inport  PortDimensions=1
  C+ : Inport  Port=2  PortDimensions=1
  Constant : Constant  Value=-1
  Logical Operator : Logic  Operator=NOT  AllPortsSameDT=off  OutDataTypeStr=boolean
  Logical Operator1 : Logic  Operator=NOT  AllPortsSameDT=off  OutDataTypeStr=boolean
  Mux : Mux
  Product : Product
  Relational Operator1 : RelationalOperator  OutDataTypeStr=boolean  InputSameDT=off
  Relational Operator2 : RelationalOperator  OutDataTypeStr=boolean  InputSameDT=off
  Result : Outport
  wires:
  Logical Operator1/1 -> Mux/3
  Relational Operator1/1 -> Mux/4, Logical Operator1/1
  Mux/1 -> Result/1
  Product/1 -> Relational Operator1/2
  Constant/1 -> Product/2
  Logical Operator/1 -> Mux/2
  Relational Operator2/1 -> Mux/1, Logical Operator/1
  Modul/1 -> Relational Operator2/1, Relational Operator1/1
  C+/1 -> Product/1, Relational Operator2/2

== system three_H_bridge/发波4/单级倍频调制 ==
  note: 1
  Modul : Inport  PortDimensions=1
  C+ : Inport  Port=2  PortDimensions=1
  Constant : Constant  Value=-1
  Logical Operator : Logic  Operator=NOT  AllPortsSameDT=off  OutDataTypeStr=boolean
  Logical Operator1 : Logic  Operator=NOT  AllPortsSameDT=off  OutDataTypeStr=boolean
  Mux : Mux
  Product : Product
  Relational Operator1 : RelationalOperator  OutDataTypeStr=boolean  InputSameDT=off
  Relational Operator2 : RelationalOperator  OutDataTypeStr=boolean  InputSameDT=off
  Result : Outport
  wires:
  C+/1 -> Relational Operator2/2, Product/1
  Modul/1 -> Relational Operator1/1, Relational Operator2/1
  Relational Operator2/1 -> Logical Operator/1, Mux/1
  Logical Operator/1 -> Mux/2
  Constant/1 -> Product/2
  Product/1 -> Relational Operator1/2
  Mux/1 -> Result/1
  Relational Operator1/1 -> Logical Operator1/1, Mux/4
  Logical Operator1/1 -> Mux/3

== system three_H_bridge/发波4/单级倍频调制1 ==
  note: 1
  Modul : Inport  PortDimensions=1
  C+ : Inport  Port=2  PortDimensions=1
  Constant : Constant  Value=-1
  Logical Operator : Logic  Operator=NOT  AllPortsSameDT=off  OutDataTypeStr=boolean
  Logical Operator1 : Logic  Operator=NOT  AllPortsSameDT=off  OutDataTypeStr=boolean
  Mux : Mux
  Product : Product
  Relational Operator1 : RelationalOperator  OutDataTypeStr=boolean  InputSameDT=off
  Relational Operator2 : RelationalOperator  OutDataTypeStr=boolean  InputSameDT=off
  Result : Outport
  wires:
  Logical Operator1/1 -> Mux/3
  Relational Operator1/1 -> Mux/4, Logical Operator1/1
  Mux/1 -> Result/1
  Product/1 -> Relational Operator1/2
  Constant/1 -> Product/2
  Logical Operator/1 -> Mux/2
  Relational Operator2/1 -> Mux/1, Logical Operator/1
  Modul/1 -> Relational Operator2/1, Relational Operator1/1
  C+/1 -> Product/1, Relational Operator2/2

== system three_H_bridge/发波4/单级倍频调制2 ==
  note: 1
  Modul : Inport  PortDimensions=1
  C+ : Inport  Port=2  PortDimensions=1
  Constant : Constant  Value=-1
  Logical Operator : Logic  Operator=NOT  AllPortsSameDT=off  OutDataTypeStr=boolean
  Logical Operator1 : Logic  Operator=NOT  AllPortsSameDT=off  OutDataTypeStr=boolean
  Mux : Mux
  Product : Product
  Relational Operator1 : RelationalOperator  OutDataTypeStr=boolean  InputSameDT=off
  Relational Operator2 : RelationalOperator  OutDataTypeStr=boolean  InputSameDT=off
  Result : Outport
  wires:
  C+/1 -> Relational Operator2/2, Product/1
  Modul/1 -> Relational Operator1/1, Relational Operator2/1
  Relational Operator2/1 -> Logical Operator/1, Mux/1
  Logical Operator/1 -> Mux/2
  Constant/1 -> Product/2
  Product/1 -> Relational Operator1/2
  Mux/1 -> Result/1
  Relational Operator1/1 -> Logical Operator1/1, Mux/4
  Logical Operator1/1 -> Mux/3

== system three_H_bridge/发波5/单级倍频调制 ==
  note: 1
  Modul : Inport  PortDimensions=1
  C+ : Inport  Port=2  PortDimensions=1
  Constant : Constant  Value=-1
  Logical Operator : Logic  Operator=NOT  AllPortsSameDT=off  OutDataTypeStr=boolean
  Logical Operator1 : Logic  Operator=NOT  AllPortsSameDT=off  OutDataTypeStr=boolean
  Mux : Mux
  Product : Product
  Relational Operator1 : RelationalOperator  OutDataTypeStr=boolean  InputSameDT=off
  Relational Operator2 : RelationalOperator  OutDataTypeStr=boolean  InputSameDT=off
  Result : Outport
  wires:
  Logical Operator1/1 -> Mux/3
  Relational Operator1/1 -> Mux/4, Logical Operator1/1
  Mux/1 -> Result/1
  Product/1 -> Relational Operator1/2
  Constant/1 -> Product/2
  Logical Operator/1 -> Mux/2
  Relational Operator2/1 -> Mux/1, Logical Operator/1
  Modul/1 -> Relational Operator2/1, Relational Operator1/1
  C+/1 -> Product/1, Relational Operator2/2

== system three_H_bridge/发波5/单级倍频调制1 ==
  note: 1
  Modul : Inport  PortDimensions=1
  C+ : Inport  Port=2  PortDimensions=1
  Constant : Constant  Value=-1
  Logical Operator : Logic  Operator=NOT  AllPortsSameDT=off  OutDataTypeStr=boolean
  Logical Operator1 : Logic  Operator=NOT  AllPortsSameDT=off  OutDataTypeStr=boolean
  Mux : Mux
  Product : Product
  Relational Operator1 : RelationalOperator  OutDataTypeStr=boolean  InputSameDT=off
  Relational Operator2 : RelationalOperator  OutDataTypeStr=boolean  InputSameDT=off
  Result : Outport
  wires:
  C+/1 -> Relational Operator2/2, Product/1
  Modul/1 -> Relational Operator1/1, Relational Operator2/1
  Relational Operator2/1 -> Logical Operator/1, Mux/1
  Logical Operator/1 -> Mux/2
  Constant/1 -> Product/2
  Product/1 -> Relational Operator1/2
  Mux/1 -> Result/1
  Relational Operator1/1 -> Logical Operator1/1, Mux/4
  Logical Operator1/1 -> Mux/3

== system three_H_bridge/发波5/单级倍频调制2 ==
  note: 1
  Modul : Inport  PortDimensions=1
  C+ : Inport  Port=2  PortDimensions=1
  Constant : Constant  Value=-1
  Logical Operator : Logic  Operator=NOT  AllPortsSameDT=off  OutDataTypeStr=boolean
  Logical Operator1 : Logic  Operator=NOT  AllPortsSameDT=off  OutDataTypeStr=boolean
  Mux : Mux
  Product : Product
  Relational Operator1 : RelationalOperator  OutDataTypeStr=boolean  InputSameDT=off
  Relational Operator2 : RelationalOperator  OutDataTypeStr=boolean  InputSameDT=off
  Result : Outport
  wires:
  Logical Operator1/1 -> Mux/3
  Relational Operator1/1 -> Mux/4, Logical Operator1/1
  Mux/1 -> Result/1
  Product/1 -> Relational Operator1/2
  Constant/1 -> Product/2
  Logical Operator/1 -> Mux/2
  Relational Operator2/1 -> Mux/1, Logical Operator/1
  Modul/1 -> Relational Operator2/1, Relational Operator1/1
  C+/1 -> Product/1, Relational Operator2/2

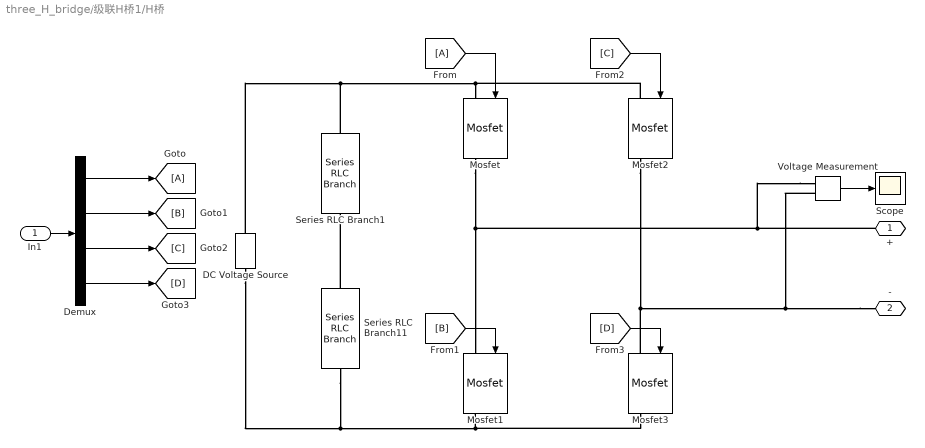
== system three_H_bridge/级联H桥1/H桥 ==
  In1 : Inport
  DC Voltage Source : spsDCVoltageSourceLib/DC Voltage Source  Amplitude=650  Measurements=None
  Demux : Demux
  From : From
  Goto : Goto
  Mosfet{,1..3} (4 alike) : spsMosfetLib/Mosfet  Ron=0.1  Lon=0  Rd=0.01  Vfd=0  IC=0  Rs=1e5  Cs=inf  Measurements=on
  Scope : Scope
  Series RLC Branch1 : spsSeriesRLCBranchLib/Series RLC Branch  LConnTagsString=__new0  RConnTagsString=__new0  BranchType=RC  Resistance=0.001  Inductance=1e-3  SetiL0=off  InitialCurrent=0  Capacitance=60e-6  Setx0=off  InitialVoltage=0  Measurements=None
  Series RLC Branch11 : spsSeriesRLCBranchLib/Series RLC Branch  LConnTagsString=__new0  RConnTagsString=__new0  BranchType=RC  Resistance=0.001  Inductance=1e-3  SetiL0=off  InitialCurrent=0  Capacitance=60e-6  Setx0=off  InitialVoltage=0  Measurements=None
  Voltage Measurement : spsVoltageMeasurementLib/Voltage Measurement  PhasorSimulation=off  OutputType=Complex  PSBequivalent=0
  + : PMIOPort  Side=Right
  - : PMIOPort  Port=2  Side=Right
  wires:
  Voltage Measurement/1 -> Scope/1
  [D] -> Mosfet3/1
  [C] -> Mosfet2/1
  [B] -> Mosfet1/1
  From/1 -> Mosfet/1
  Demux/4 -> [D]
  Demux/3 -> [C]
  Demux/2 -> [B]
  Demux/1 -> Goto/1
  In1/1 -> Demux/1
  connections:
  Series RLC Branch11/LConn1 -- Series RLC Branch1/RConn1
  Mosfet1/RConn1 -- Mosfet3/RConn1 -- Series RLC Branch11/RConn1 -- DC Voltage Source/LConn1
  Voltage Measurement/LConn1 -- Mosfet/RConn1 -- Mosfet1/LConn1 -- +/RConn1
  -/RConn1 -- Voltage Measurement/LConn2 -- Mosfet3/LConn1 -- Mosfet2/RConn1
  Series RLC Branch1/LConn1 -- Mosfet/LConn1 -- Mosfet2/LConn1 -- DC Voltage Source/RConn1

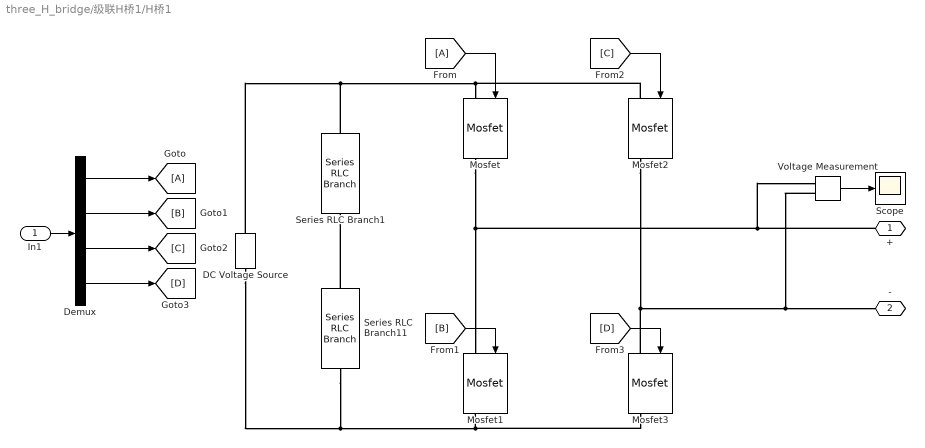
== system three_H_bridge/级联H桥1/H桥1 ==
  In1 : Inport
  DC Voltage Source : spsDCVoltageSourceLib/DC Voltage Source  Amplitude=650  Measurements=None
  Demux : Demux
  From : From
  Goto : Goto
  Mosfet{,1..3} (4 alike) : spsMosfetLib/Mosfet  Ron=0.1  Lon=0  Rd=0.01  Vfd=0  IC=0  Rs=1e5  Cs=inf  Measurements=on
  Scope : Scope
  Series RLC Branch1 : spsSeriesRLCBranchLib/Series RLC Branch  LConnTagsString=__new0  RConnTagsString=__new0  BranchType=RC  Resistance=0.001  Inductance=1e-3  SetiL0=off  InitialCurrent=0  Capacitance=60e-6  Setx0=off  InitialVoltage=0  Measurements=None
  Series RLC Branch11 : spsSeriesRLCBranchLib/Series RLC Branch  LConnTagsString=__new0  RConnTagsString=__new0  BranchType=RC  Resistance=0.001  Inductance=1e-3  SetiL0=off  InitialCurrent=0  Capacitance=60e-6  Setx0=off  InitialVoltage=0  Measurements=None
  Voltage Measurement : spsVoltageMeasurementLib/Voltage Measurement  PhasorSimulation=off  OutputType=Complex  PSBequivalent=0
  + : PMIOPort  Side=Right
  - : PMIOPort  Port=2  Side=Right
  wires:
  In1/1 -> Demux/1
  Demux/1 -> Goto/1
  Demux/2 -> [B]
  Demux/3 -> [C]
  Demux/4 -> [D]
  From/1 -> Mosfet/1
  [B] -> Mosfet1/1
  [C] -> Mosfet2/1
  [D] -> Mosfet3/1
  Voltage Measurement/1 -> Scope/1
  connections:
  DC Voltage Source/RConn1 -- Mosfet2/LConn1 -- Mosfet/LConn1 -- Series RLC Branch1/LConn1
  Mosfet2/RConn1 -- Mosfet3/LConn1 -- Voltage Measurement/LConn2 -- -/RConn1
  +/RConn1 -- Mosfet1/LConn1 -- Mosfet/RConn1 -- Voltage Measurement/LConn1
  DC Voltage Source/LConn1 -- Series RLC Branch11/RConn1 -- Mosfet3/RConn1 -- Mosfet1/RConn1
  Series RLC Branch11/LConn1 -- Series RLC Branch1/RConn1

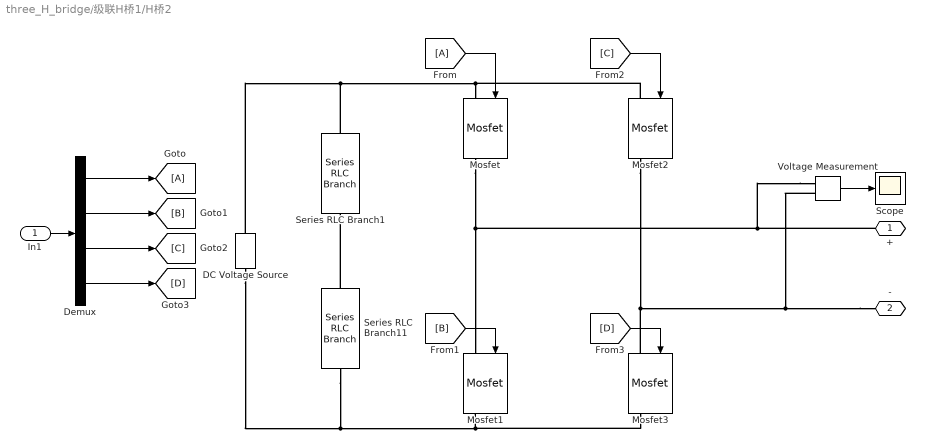
== system three_H_bridge/级联H桥1/H桥2 ==
  In1 : Inport
  DC Voltage Source : spsDCVoltageSourceLib/DC Voltage Source  Amplitude=650  Measurements=None
  Demux : Demux
  From : From
  Goto : Goto
  Mosfet{,1..3} (4 alike) : spsMosfetLib/Mosfet  Ron=0.1  Lon=0  Rd=0.01  Vfd=0  IC=0  Rs=1e5  Cs=inf  Measurements=on
  Scope : Scope
  Series RLC Branch1 : spsSeriesRLCBranchLib/Series RLC Branch  LConnTagsString=__new0  RConnTagsString=__new0  BranchType=RC  Resistance=0.001  Inductance=1e-3  SetiL0=off  InitialCurrent=0  Capacitance=60e-6  Setx0=off  InitialVoltage=0  Measurements=None
  Series RLC Branch11 : spsSeriesRLCBranchLib/Series RLC Branch  LConnTagsString=__new0  RConnTagsString=__new0  BranchType=RC  Resistance=0.001  Inductance=1e-3  SetiL0=off  InitialCurrent=0  Capacitance=60e-6  Setx0=off  InitialVoltage=0  Measurements=None
  Voltage Measurement : spsVoltageMeasurementLib/Voltage Measurement  PhasorSimulation=off  OutputType=Complex  PSBequivalent=0
  + : PMIOPort  Side=Right
  - : PMIOPort  Port=2  Side=Right
  wires:
  Voltage Measurement/1 -> Scope/1
  [D] -> Mosfet3/1
  [C] -> Mosfet2/1
  [B] -> Mosfet1/1
  From/1 -> Mosfet/1
  Demux/4 -> [D]
  Demux/3 -> [C]
  Demux/2 -> [B]
  Demux/1 -> Goto/1
  In1/1 -> Demux/1
  connections:
  Series RLC Branch11/LConn1 -- Series RLC Branch1/RConn1
  Mosfet1/RConn1 -- Mosfet3/RConn1 -- Series RLC Branch11/RConn1 -- DC Voltage Source/LConn1
  Voltage Measurement/LConn1 -- Mosfet/RConn1 -- Mosfet1/LConn1 -- +/RConn1
  -/RConn1 -- Voltage Measurement/LConn2 -- Mosfet3/LConn1 -- Mosfet2/RConn1
  Series RLC Branch1/LConn1 -- Mosfet/LConn1 -- Mosfet2/LConn1 -- DC Voltage Source/RConn1

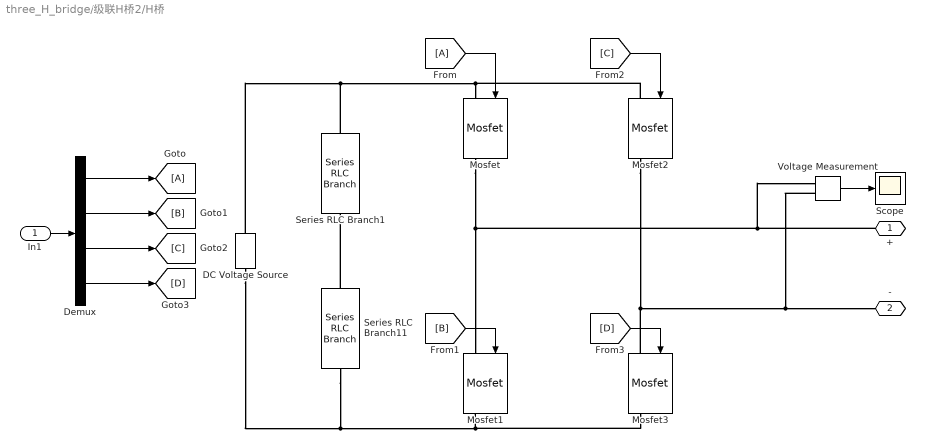
== system three_H_bridge/级联H桥2/H桥 ==
  In1 : Inport
  DC Voltage Source : spsDCVoltageSourceLib/DC Voltage Source  Amplitude=650  Measurements=None
  Demux : Demux
  From : From
  Goto : Goto
  Mosfet{,1..3} (4 alike) : spsMosfetLib/Mosfet  Ron=0.1  Lon=0  Rd=0.01  Vfd=0  IC=0  Rs=1e5  Cs=inf  Measurements=on
  Scope : Scope
  Series RLC Branch1 : spsSeriesRLCBranchLib/Series RLC Branch  LConnTagsString=__new0  RConnTagsString=__new0  BranchType=RC  Resistance=0.001  Inductance=1e-3  SetiL0=off  InitialCurrent=0  Capacitance=60e-6  Setx0=off  InitialVoltage=0  Measurements=None
  Series RLC Branch11 : spsSeriesRLCBranchLib/Series RLC Branch  LConnTagsString=__new0  RConnTagsString=__new0  BranchType=RC  Resistance=0.001  Inductance=1e-3  SetiL0=off  InitialCurrent=0  Capacitance=60e-6  Setx0=off  InitialVoltage=0  Measurements=None
  Voltage Measurement : spsVoltageMeasurementLib/Voltage Measurement  PhasorSimulation=off  OutputType=Complex  PSBequivalent=0
  + : PMIOPort  Side=Right
  - : PMIOPort  Port=2  Side=Right
  wires:
  In1/1 -> Demux/1
  Demux/1 -> Goto/1
  Demux/2 -> [B]
  Demux/3 -> [C]
  Demux/4 -> [D]
  From/1 -> Mosfet/1
  [B] -> Mosfet1/1
  [C] -> Mosfet2/1
  [D] -> Mosfet3/1
  Voltage Measurement/1 -> Scope/1
  connections:
  DC Voltage Source/RConn1 -- Mosfet2/LConn1 -- Mosfet/LConn1 -- Series RLC Branch1/LConn1
  Mosfet2/RConn1 -- Mosfet3/LConn1 -- Voltage Measurement/LConn2 -- -/RConn1
  +/RConn1 -- Mosfet1/LConn1 -- Mosfet/RConn1 -- Voltage Measurement/LConn1
  DC Voltage Source/LConn1 -- Series RLC Branch11/RConn1 -- Mosfet3/RConn1 -- Mosfet1/RConn1
  Series RLC Branch11/LConn1 -- Series RLC Branch1/RConn1

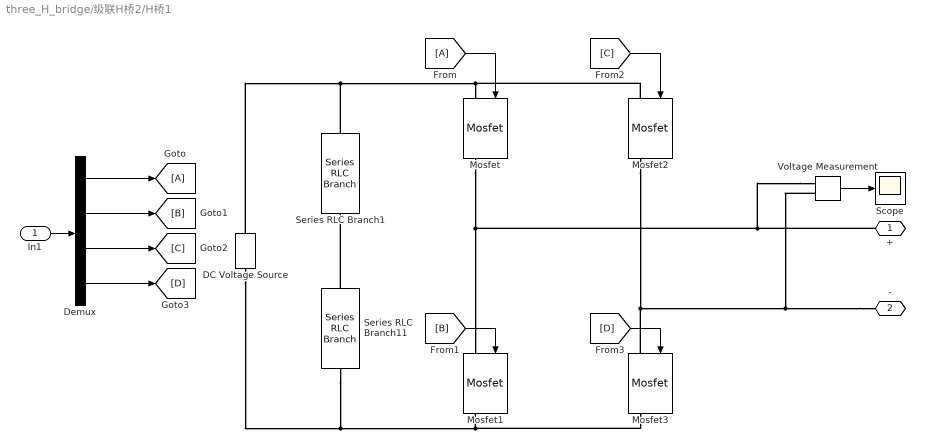
== system three_H_bridge/级联H桥2/H桥1 ==
  In1 : Inport
  DC Voltage Source : spsDCVoltageSourceLib/DC Voltage Source  Amplitude=650  Measurements=None
  Demux : Demux
  From : From
  Goto : Goto
  Mosfet{,1..3} (4 alike) : spsMosfetLib/Mosfet  Ron=0.1  Lon=0  Rd=0.01  Vfd=0  IC=0  Rs=1e5  Cs=inf  Measurements=on
  Scope : Scope
  Series RLC Branch1 : spsSeriesRLCBranchLib/Series RLC Branch  LConnTagsString=__new0  RConnTagsString=__new0  BranchType=RC  Resistance=0.001  Inductance=1e-3  SetiL0=off  InitialCurrent=0  Capacitance=60e-6  Setx0=off  InitialVoltage=0  Measurements=None
  Series RLC Branch11 : spsSeriesRLCBranchLib/Series RLC Branch  LConnTagsString=__new0  RConnTagsString=__new0  BranchType=RC  Resistance=0.001  Inductance=1e-3  SetiL0=off  InitialCurrent=0  Capacitance=60e-6  Setx0=off  InitialVoltage=0  Measurements=None
  Voltage Measurement : spsVoltageMeasurementLib/Voltage Measurement  PhasorSimulation=off  OutputType=Complex  PSBequivalent=0
  + : PMIOPort  Side=Right
  - : PMIOPort  Port=2  Side=Right
  wires:
  Voltage Measurement/1 -> Scope/1
  [D] -> Mosfet3/1
  [C] -> Mosfet2/1
  [B] -> Mosfet1/1
  From/1 -> Mosfet/1
  Demux/4 -> [D]
  Demux/3 -> [C]
  Demux/2 -> [B]
  Demux/1 -> Goto/1
  In1/1 -> Demux/1
  connections:
  Series RLC Branch11/LConn1 -- Series RLC Branch1/RConn1
  Mosfet1/RConn1 -- Mosfet3/RConn1 -- Series RLC Branch11/RConn1 -- DC Voltage Source/LConn1
  Voltage Measurement/LConn1 -- Mosfet/RConn1 -- Mosfet1/LConn1 -- +/RConn1
  -/RConn1 -- Voltage Measurement/LConn2 -- Mosfet3/LConn1 -- Mosfet2/RConn1
  Series RLC Branch1/LConn1 -- Mosfet/LConn1 -- Mosfet2/LConn1 -- DC Voltage Source/RConn1

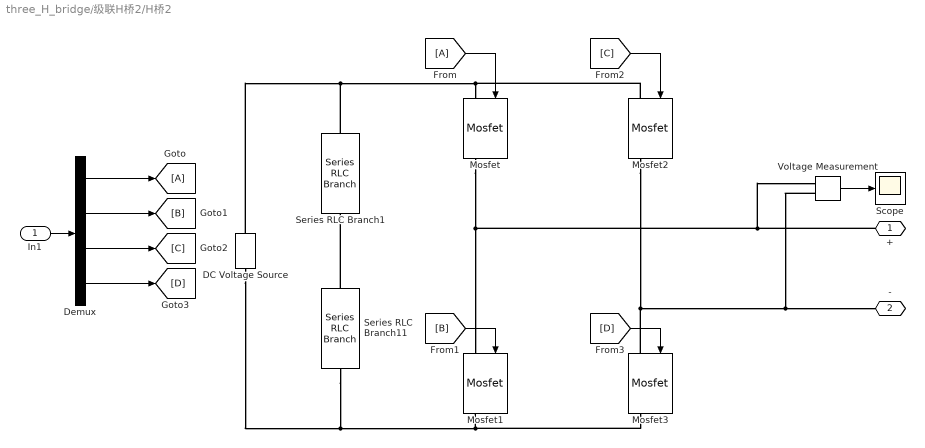
== system three_H_bridge/级联H桥2/H桥2 ==
  In1 : Inport
  DC Voltage Source : spsDCVoltageSourceLib/DC Voltage Source  Amplitude=650  Measurements=None
  Demux : Demux
  From : From
  Goto : Goto
  Mosfet{,1..3} (4 alike) : spsMosfetLib/Mosfet  Ron=0.1  Lon=0  Rd=0.01  Vfd=0  IC=0  Rs=1e5  Cs=inf  Measurements=on
  Scope : Scope
  Series RLC Branch1 : spsSeriesRLCBranchLib/Series RLC Branch  LConnTagsString=__new0  RConnTagsString=__new0  BranchType=RC  Resistance=0.001  Inductance=1e-3  SetiL0=off  InitialCurrent=0  Capacitance=60e-6  Setx0=off  InitialVoltage=0  Measurements=None
  Series RLC Branch11 : spsSeriesRLCBranchLib/Series RLC Branch  LConnTagsString=__new0  RConnTagsString=__new0  BranchType=RC  Resistance=0.001  Inductance=1e-3  SetiL0=off  InitialCurrent=0  Capacitance=60e-6  Setx0=off  InitialVoltage=0  Measurements=None
  Voltage Measurement : spsVoltageMeasurementLib/Voltage Measurement  PhasorSimulation=off  OutputType=Complex  PSBequivalent=0
  + : PMIOPort  Side=Right
  - : PMIOPort  Port=2  Side=Right
  wires:
  In1/1 -> Demux/1
  Demux/1 -> Goto/1
  Demux/2 -> [B]
  Demux/3 -> [C]
  Demux/4 -> [D]
  From/1 -> Mosfet/1
  [B] -> Mosfet1/1
  [C] -> Mosfet2/1
  [D] -> Mosfet3/1
  Voltage Measurement/1 -> Scope/1
  connections:
  DC Voltage Source/RConn1 -- Mosfet2/LConn1 -- Mosfet/LConn1 -- Series RLC Branch1/LConn1
  Mosfet2/RConn1 -- Mosfet3/LConn1 -- Voltage Measurement/LConn2 -- -/RConn1
  +/RConn1 -- Mosfet1/LConn1 -- Mosfet/RConn1 -- Voltage Measurement/LConn1
  DC Voltage Source/LConn1 -- Series RLC Branch11/RConn1 -- Mosfet3/RConn1 -- Mosfet1/RConn1
  Series RLC Branch11/LConn1 -- Series RLC Branch1/RConn1

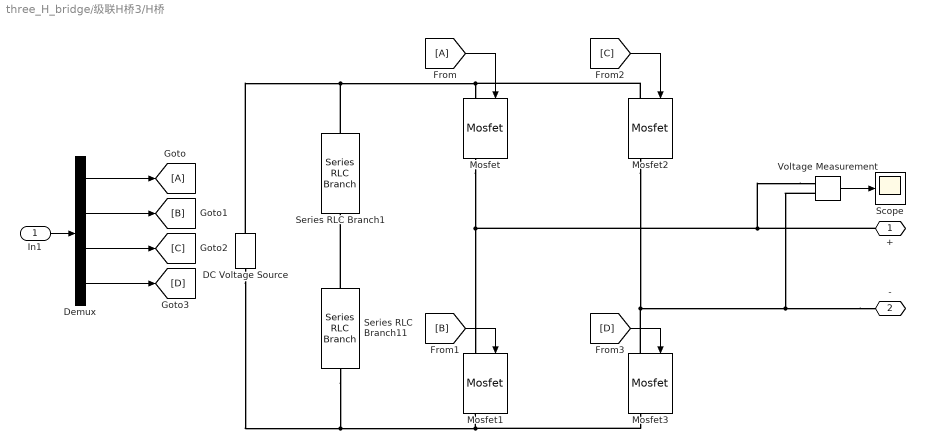
== system three_H_bridge/级联H桥3/H桥 ==
  In1 : Inport
  DC Voltage Source : spsDCVoltageSourceLib/DC Voltage Source  Amplitude=650  Measurements=None
  Demux : Demux
  From : From
  Goto : Goto
  Mosfet{,1..3} (4 alike) : spsMosfetLib/Mosfet  Ron=0.1  Lon=0  Rd=0.01  Vfd=0  IC=0  Rs=1e5  Cs=inf  Measurements=on
  Scope : Scope
  Series RLC Branch1 : spsSeriesRLCBranchLib/Series RLC Branch  LConnTagsString=__new0  RConnTagsString=__new0  BranchType=RC  Resistance=0.001  Inductance=1e-3  SetiL0=off  InitialCurrent=0  Capacitance=60e-6  Setx0=off  InitialVoltage=0  Measurements=None
  Series RLC Branch11 : spsSeriesRLCBranchLib/Series RLC Branch  LConnTagsString=__new0  RConnTagsString=__new0  BranchType=RC  Resistance=0.001  Inductance=1e-3  SetiL0=off  InitialCurrent=0  Capacitance=60e-6  Setx0=off  InitialVoltage=0  Measurements=None
  Voltage Measurement : spsVoltageMeasurementLib/Voltage Measurement  PhasorSimulation=off  OutputType=Complex  PSBequivalent=0
  + : PMIOPort  Side=Right
  - : PMIOPort  Port=2  Side=Right
  wires:
  Voltage Measurement/1 -> Scope/1
  [D] -> Mosfet3/1
  [C] -> Mosfet2/1
  [B] -> Mosfet1/1
  From/1 -> Mosfet/1
  Demux/4 -> [D]
  Demux/3 -> [C]
  Demux/2 -> [B]
  Demux/1 -> Goto/1
  In1/1 -> Demux/1
  connections:
  Series RLC Branch11/LConn1 -- Series RLC Branch1/RConn1
  Mosfet1/RConn1 -- Mosfet3/RConn1 -- Series RLC Branch11/RConn1 -- DC Voltage Source/LConn1
  Voltage Measurement/LConn1 -- Mosfet/RConn1 -- Mosfet1/LConn1 -- +/RConn1
  -/RConn1 -- Voltage Measurement/LConn2 -- Mosfet3/LConn1 -- Mosfet2/RConn1
  Series RLC Branch1/LConn1 -- Mosfet/LConn1 -- Mosfet2/LConn1 -- DC Voltage Source/RConn1
